simulink model "Hausuebung_Simulink"  (R2020b)
settings: Solver=ode45  StartTime=0.0  StopTime=1  RelTol=1e-10  AbsTol=1e-10
settings Model: Creator=Schar  LastModifiedBy=Schar

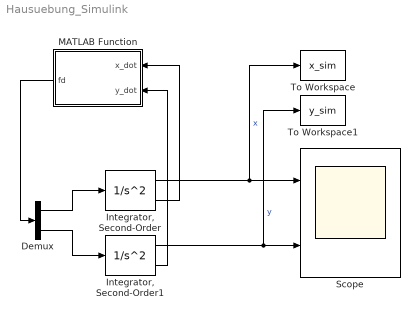
== system Hausuebung_Simulink ==
  Demux : Demux  Outputs=2
  "Integrator, Second-Order" : SecondOrderIntegrator  ICX=x0  ICDXDT=vx_0
  "Integrator, Second-Order1" : SecondOrderIntegrator  ICX=y0  ICDXDT=vy_0
  MATLAB Function : MATLAB Function  TreatAsAtomicUnit=on
  Scope : Scope  NumInputPorts=2
  To Workspace : ToWorkspace  VariableName=x_sim  SaveFormat=Timeseries  SampleTime=-1
  To Workspace1 : ToWorkspace  VariableName=y_sim  SaveFormat=Timeseries  SampleTime=-1
  wires:
  Demux/1 -> "Integrator, Second-Order"/1
  "Integrator, Second-Order"/2 -> MATLAB Function/1(x_dot)
  "Integrator, Second-Order"/1 -> To Workspace/1, Scope/1  "x"
  "Integrator, Second-Order1"/2 -> MATLAB Function/2(y_dot)
  "Integrator, Second-Order1"/1 -> To Workspace1/1, Scope/2  "y"
  MATLAB Function/1(fd) -> Demux/1
  Demux/2 -> "Integrator, Second-Order1"/1

== matlab function Hausuebung_Simulink/MATLAB Function ==
  data: x_dot input; y_dot input; fd output; par parameter
function fd = fcn(x_dot, y_dot, par)

m_Ball = par.m_Ball;
g = par.g;
cw = par.cw;
d_Ball = par.d_Ball;
rho = par.rho;


fdx = -((1/8)*rho*d_Ball^2*pi*cw*sqrt(x_dot^2+y_dot^2)*x_dot)/m_Ball;
fdy = -(((1/8)*rho*d_Ball^2*pi*cw*sqrt(x_dot^2+y_dot^2)*y_dot)/m_Ball)-g;
fd = [fdx, fdy];
